simulink library "xps_library"  (R2021a)
settings: Solver=VariableStepAuto  StartTime=0.0  StopTime=10.0  RelTol=1e-3
undefined symbols (not defined in the file or in its folder): ip_name, lib_path
libraries: xbsIndex_r4 x2626, casper_library_flow_control x68, simulink x52, $bdroot x9, casper_library_misc x9
(part 5 of 33)

== system xps_library/Platforms ==
  ADM_PCIE_9H7 : Subsystem  Tag=xps:xsg  mask(xsg core config){hw_sys=ADM_PCIE_9H7:xcvu37p, clk_src=sys_clk, clk_rate=100, use_microblaze=off, use_pr=on, pr_template='', sample_period=1, synthesis_tool=XST}
      mask prompts: hw_sys "Hardware Platform"; clk_src "User IP Clock source"; clk_rate "User IP Clock Rate (MHz)"; use_microblaze "Use Microblaze controller?"; use_pr "Use PCIe Partial Reconfiguration"; sample_period "Sample Period"; synthesis_tool "Synthesis Tool:"
      mask help:
      | The XSG Core Config block is used to configure the System Generator design
      | for the casper_xps toolflow. Settings here are used to configure the
      | Xilinx System Generator block parameters automatically, and control toolflow
      | script  execution. It needs to be at the top level of all designs being compiled
      | with the casper_xps toolflow.
      mask init:
      | xps_xsg_adm_pcie_9h7_conf_mask;
      mask Help: eval('xlWeb([getenv(''MLIB_ROOT''), ''\doc\html\sys_xsg_core_config\sys_xsg_core_config.html''])')
      mask TypeOptions hw_sys: ADM_PCIE_9H7:xcvu37p
      mask TypeOptions clk_src: sys_clk | dts_clk
      mask TypeOptions synthesis_tool: Leonardo Spectrum | Synplify | Synplify Pro | XST
      mask Display: fprintf(['ADM\nPCIE_9H7']);
  AU280 : Subsystem  Tag=xps:xsg  mask(xsg core config){hw_sys=AU280:xcu280, clk_src=sys_clk, clk_rate=156.25, sample_period=1, synthesis_tool=XST}
      mask prompts: hw_sys "Hardware Platform"; clk_src "User IP Clock source"; clk_rate "User IP Clock Rate (MHz)"; sample_period "Sample Period"; synthesis_tool "Synthesis Tool:"
      mask help:
      | The XSG Core Config block is used to configure the System Generator design
      | for the casper_xps toolflow. Settings here are used to configure the
      | Xilinx System Generator block parameters automatically, and control toolflow
      | script  execution. It needs to be at the top level of all designs being compiled
      | with the casper_xps toolflow.
      mask init:
      | xps_xsg_au280_conf_mask;
      mask Help: eval('xlWeb([getenv(''MLIB_ROOT''), ''\doc\html\sys_xsg_core_config\sys_xsg_core_config.html''])')
      mask TypeOptions hw_sys: AU280:xcu280
      mask TypeOptions clk_src: sys_clk | aux_clk
      mask TypeOptions synthesis_tool: Leonardo Spectrum | Synplify | Synplify Pro | XST
      mask Display: fprintf(['ALVEO_U280']);
  AU50 : Subsystem  Tag=xps:xsg  mask(xsg core config){hw_sys=AU50:xcu50, clk_src=sys_clk, clk_rate=156.25, sample_period=1, synthesis_tool=XST}
      mask prompts: hw_sys "Hardware Platform"; clk_src "User IP Clock source"; clk_rate "User IP Clock Rate (MHz)"; sample_period "Sample Period"; synthesis_tool "Synthesis Tool:"
      mask help:
      | The XSG Core Config block is used to configure the System Generator design
      | for the casper_xps toolflow. Settings here are used to configure the
      | Xilinx System Generator block parameters automatically, and control toolflow
      | script  execution. It needs to be at the top level of all designs being compiled
      | with the casper_xps toolflow.
      mask init:
      | xps_xsg_au50_conf_mask;
      mask Help: eval('xlWeb([getenv(''MLIB_ROOT''), ''\doc\html\sys_xsg_core_config\sys_xsg_core_config.html''])')
      mask TypeOptions hw_sys: AU50:xcu50
      mask TypeOptions clk_src: sys_clk | aux_clk
      mask TypeOptions synthesis_tool: Leonardo Spectrum | Synplify | Synplify Pro | XST
      mask Display: fprintf(['ALVEO_U50']);
  CASIA_K7 : Subsystem  Tag=xps:xsg  AncestorBlock=xps_merge/Platforms/CASIA_K7  mask(xsg core config){hw_sys=CASIA_K7:xc7k325t, clk_src=sys_clk, clk_rate=100, use_microblaze=on, sample_period=1, synthesis_tool=XST}
      mask prompts: hw_sys "Hardware Platform"; clk_src "User IP Clock source"; clk_rate "User IP Clock Rate (MHz)"; use_microblaze "Use Microblaze controller?"; sample_period "Sample Period"; synthesis_tool "Synthesis Tool:"
      mask help:
      | The XSG Core Config block is used to configure the System Generator design
      | for the casper_xps toolflow. Settings here are used to configure the
      | Xilinx System Generator block parameters automatically, and control toolflow
      | script  execution. It needs to be at the top level of all designs being compiled
      | with the casper_xps toolflow.
      mask init:
      | xps_xsg_casia_k7_conf_mask;
      mask Help: eval('xlWeb([getenv(''MLIB_ROOT''), ''\doc\html\sys_xsg_core_config\sys_xsg_core_config.html''])')
      mask TypeOptions hw_sys: CASIA_K7:xc7k325t
      mask TypeOptions clk_src: sys_clk | clk_250MHz | adc_clk
      mask TypeOptions synthesis_tool: Leonardo Spectrum | Synplify | Synplify Pro | XST
      mask Display: fprintf(['CASIA_K7']);
  CASIA_K7_21CMA : Subsystem  Tag=xps:xsg  AncestorBlock=xps_merge/Platforms/CASIA_K7_21CMA  mask(xsg core config){hw_sys=CASIA_K7_21CMA:xc7k325t, clk_src=sys_clk, clk_rate=100, use_microblaze=on, sample_period=1, synthesis_tool=XST}
      mask prompts: hw_sys "Hardware Platform"; clk_src "User IP Clock source"; clk_rate "User IP Clock Rate (MHz)"; use_microblaze "Use Microblaze controller?"; sample_period "Sample Period"; synthesis_tool "Synthesis Tool:"
      mask help:
      | The XSG Core Config block is used to configure the System Generator design
      | for the casper_xps toolflow. Settings here are used to configure the
      | Xilinx System Generator block parameters automatically, and control toolflow
      | script  execution. It needs to be at the top level of all designs being compiled
      | with the casper_xps toolflow.
      mask init:
      | xps_xsg_casia_k7_21cma_conf_mask;
      mask Help: eval('xlWeb([getenv(''MLIB_ROOT''), ''\doc\html\sys_xsg_core_config\sys_xsg_core_config.html''])')
      mask TypeOptions hw_sys: CASIA_K7_21CMA:xc7k325t
      mask TypeOptions clk_src: sys_clk | clk_250MHz | adc_clk
      mask TypeOptions synthesis_tool: Leonardo Spectrum | Synplify | Synplify Pro | XST
      mask Display: fprintf(['CASIA_K7_21CMA']);
  HTG9200 : Subsystem  Tag=xps:xsg  mask(xsg core config){hw_sys=HTG9200:xcvu13p, clk_src=sys_clk, clk_rate=100, use_microblaze=on, sample_period=1, synthesis_tool=XST}
      mask prompts: hw_sys "Hardware Platform"; clk_src "User IP Clock source"; clk_rate "User IP Clock Rate (MHz)"; use_microblaze "Use Microblaze controller?"; sample_period "Sample Period"; synthesis_tool "Synthesis Tool:"
      mask help:
      | The XSG Core Config block is used to configure the System Generator design
      | for the casper_xps toolflow. Settings here are used to configure the
      | Xilinx System Generator block parameters automatically, and control toolflow
      | script  execution. It needs to be at the top level of all designs being compiled
      | with the casper_xps toolflow.
      mask init:
      | xps_xsg_htg9200_conf_mask;
      mask Help: eval('xlWeb([getenv(''MLIB_ROOT''), ''\doc\html\sys_xsg_core_config\sys_xsg_core_config.html''])')
      mask TypeOptions hw_sys: HTG9200:xcvu13p
      mask TypeOptions clk_src: sys_clk | clk_250
      mask TypeOptions synthesis_tool: Leonardo Spectrum | Synplify | Synplify Pro | XST
      mask Display: fprintf(['HTG9200']);
  HTG940 : Subsystem  Tag=xps:xsg  mask(xsg core config){hw_sys=HTG940:xcvu13p, clk_src=fmc_c_clk, clk_rate=312.5, use_microblaze=on, sample_period=1, synthesis_tool=XST}
      mask prompts: hw_sys "Hardware Platform"; clk_src "User IP Clock source"; clk_rate "User IP Clock Rate (MHz)"; use_microblaze "Use Microblaze controller?"; sample_period "Sample Period"; synthesis_tool "Synthesis Tool:"
      mask help:
      | The XSG Core Config block is used to configure the System Generator design
      | for the casper_xps toolflow. Settings here are used to configure the
      | Xilinx System Generator block parameters automatically, and control toolflow
      | script  execution. It needs to be at the top level of all designs being compiled
      | with the casper_xps toolflow.
      mask init:
      | xps_xsg_htg940_conf_mask;
      mask Help: eval('xlWeb([getenv(''MLIB_ROOT''), ''\doc\html\sys_xsg_core_config\sys_xsg_core_config.html''])')
      mask TypeOptions hw_sys: HTG940:xcvu13p
      mask TypeOptions clk_src: sys_clk | fmc_a_clk | fmc_b_clk | fmc_c_clk | fmc_d_clk | ddr_refclk
      mask TypeOptions synthesis_tool: Leonardo Spectrum | Synplify | Synplify Pro | XST
      mask Display: fprintf(['HTG940']);
  HTG_ZRF16 : Subsystem  Tag=xps:xsg  mask(xsg core config){hw_sys=htg_zrf16:xczu49dr, clk_src=sys_clk, clk_rate=100, sample_period=1, synthesis_tool=XST}
      mask prompts: hw_sys "Hardware Platform"; clk_src "User IP Clock source"; clk_rate "User IP Clock Rate (MHz)"; sample_period "Sample Period"; synthesis_tool "Synthesis Tool:"
      mask help:
      | The XSG Core Config block is used to configure the System Generator design
      | for the casper_xps toolflow. Settings here are used to configure the
      | Xilinx System Generator block parameters automatically, and control toolflow
      | script  execution. It needs to be at the top level of all designs being compiled
      | with the casper_xps toolflow.
      mask init:
      | xps_xsg_htg_zrf16_conf_mask;
      mask Help: eval('xlWeb([getenv(''MLIB_ROOT''), ''\doc\html\sys_xsg_core_config\sys_xsg_core_config.html''])')
      mask TypeOptions hw_sys: htg_zrf16:xczu29dr | htg_zrf16:xczu49dr
      mask TypeOptions clk_src: sys_clk | adc_clk | arb_clk
      mask TypeOptions synthesis_tool: Leonardo Spectrum | Synplify | Synplify Pro | XST
      mask Display: fprintf(['ZRF16']);
  MX175 : Subsystem  Tag=xps:xsg  mask(xsg core config){hw_sys=MX175:xc7vx690t, clk_src=sys_clk, clk_rate=100, use_microblaze=off, sample_period=1, synthesis_tool=XST}
      mask prompts: hw_sys "Hardware Platform"; clk_src "User IP Clock source"; clk_rate "User IP Clock Rate (MHz)"; use_microblaze "Use Microblaze controller?"; sample_period "Sample Period"; synthesis_tool "Synthesis Tool:"
      mask help:
      | The XSG Core Config block is used to configure the System Generator design
      | for the casper_xps toolflow. Settings here are used to configure the
      | Xilinx System Generator block parameters automatically, and control toolflow
      | script  execution. It needs to be at the top level of all designs being compiled
      | with the casper_xps toolflow.
      mask init:
      | xps_xsg_mx175_conf_mask;
      mask Help: eval('xlWeb([getenv(''MLIB_ROOT''), ''\doc\html\sys_xsg_core_config\sys_xsg_core_config.html''])')
      mask TypeOptions hw_sys: MX175:xc7vx690t
      mask TypeOptions clk_src: sys_clk | adc0_clk
      mask TypeOptions synthesis_tool: Leonardo Spectrum | Synplify | Synplify Pro | XST
      mask Display: fprintf(['MX175']);
  RED_PITAYA : Subsystem  Tag=xps:xsg  mask(xsg core config){hw_sys=RED_PITAYA_10:xc7z010, clk_src=sys_clk, clk_rate=125, sample_period=1, synthesis_tool=XST}
      mask prompts: hw_sys "Hardware Platform"; clk_src "User IP Clock source"; clk_rate "User IP Clock Rate (MHz)"; sample_period "Sample Period"; synthesis_tool "Synthesis Tool:"
      mask help:
      | The XSG Core Config block is used to configure the System Generator design
      | for the casper_xps toolflow. Settings here are used to configure the
      | Xilinx System Generator block parameters automatically, and control toolflow
      | script  execution. It needs to be at the top level of all designs being compiled
      | with the casper_xps toolflow.
      mask init:
      | xps_xsg_red_pitaya_conf_mask;
      mask Help: eval('xlWeb([getenv(''MLIB_ROOT''), ''\doc\html\sys_xsg_core_config\sys_xsg_core_config.html''])')
      mask TypeOptions hw_sys: RED_PITAYA_10:xc7z010 | RED_PITAYA_14:xc7z010
      mask TypeOptions clk_src: sys_clk | adc_clk
      mask Callback clk_src: xps_xsg_red_pitaya_conf_mask_callback;
      mask TypeOptions synthesis_tool: Leonardo Spectrum | Synplify | Synplify Pro | XST
      mask Display: fprintf(['RED_PITAYA']);
  RFSoC2x2 : Subsystem  Tag=xps:xsg  AncestorBlock=xps_library/Platforms/PYNQ2x2  mask(xsg core config){hw_sys=rfsoc2x2:xczu28dr, clk_src=adc_clk, clk_rate=245.76, pl_clk_rate=122.88, sample_period=1, synthesis_tool=XST}
      mask prompts: hw_sys "Hardware Platform"; clk_src "User IP Clock source"; clk_rate "User IP Clock Rate (MHz)"; pl_clk_rate "RFPLL PL Clock Rate (MHz)"; sample_period "Sample Period"; synthesis_tool "Synthesis Tool:"
      mask help:
      | The XSG Core Config block is used to configure the System Generator design
      | for the casper_xps toolflow. Settings here are used to configure the
      | Xilinx System Generator block parameters automatically, and control toolflow
      | script  execution. It needs to be at the top level of all designs being compiled
      | with the casper_xps toolflow.
      mask init:
      | xps_xsg_rfsoc2x2_conf_mask;
      mask Help: eval('xlWeb([getenv(''MLIB_ROOT''), ''\doc\html\sys_xsg_core_config\sys_xsg_core_config.html''])')
      mask TypeOptions hw_sys: rfsoc2x2:xczu28dr
      mask TypeOptions clk_src: adc_clk
      mask TypeOptions synthesis_tool: Leonardo Spectrum | Synplify | Synplify Pro | XST
      mask Display: fprintf(['RFSoC2x2']);
  RFSoC4x2 : Subsystem  Tag=xps:xsg  AncestorBlock=xps_library/Platforms/ZCU216  mask(xsg core config){hw_sys=rfsoc4x2:xczu48dr, clk_src=adc_clk, clk_rate=245.76, pl_clk_rate=122.88, sample_period=1, synthesis_tool=XST}
      mask prompts: hw_sys "Hardware Platform"; clk_src "User IP Clock source"; clk_rate "User IP Clock Rate (MHz)"; pl_clk_rate "RFPLL PL Clock Rate (MHz)"; sample_period "Sample Period"; synthesis_tool "Synthesis Tool:"
      mask help:
      | The XSG Core Config block is used to configure the System Generator design
      | for the casper_xps toolflow. Settings here are used to configure the
      | Xilinx System Generator block parameters automatically, and control toolflow
      | script  execution. It needs to be at the top level of all designs being compiled
      | with the casper_xps toolflow.
      mask init:
      | xps_xsg_rfsoc4x2_conf_mask;
      mask Help: eval('xlWeb([getenv(''MLIB_ROOT''), ''\doc\html\sys_xsg_core_config\sys_xsg_core_config.html''])')
      mask TypeOptions hw_sys: rfsoc4x2:xczu48dr
      mask TypeOptions clk_src: adc_clk
      mask TypeOptions synthesis_tool: Leonardo Spectrum | Synplify | Synplify Pro | XST
      mask Display: fprintf(['RFSoC4x2']);
  SKARAB : Subsystem  Tag=xps:xsg  mask(xsg core config){hw_sys=SKARAB:xc7vx690t, clk_src=adc_clk, clk_rate=230, sample_period=1, synthesis_tool=XST}
      mask prompts: hw_sys "Hardware Platform"; clk_src "User IP Clock source"; clk_rate "User IP Clock Rate (MHz)"; sample_period "Sample Period"; synthesis_tool "Synthesis Tool:"
      mask help:
      | The XSG Core Config block is used to configure the System Generator design
      | for the casper_xps toolflow. Settings here are used to configure the
      | Xilinx System Generator block parameters automatically, and control toolflow
      | script  execution. It needs to be at the top level of all designs being compiled
      | with the casper_xps toolflow.
      mask init:
      | xps_xsg_skarab_conf_mask;
      mask Help: eval('xlWeb([getenv(''MLIB_ROOT''), ''\doc\html\sys_xsg_core_config\sys_xsg_core_config.html''])')
      mask TypeOptions hw_sys: SKARAB:xc7vx690t
      mask TypeOptions clk_src: sys_clk | adc_clk | aux_clk
      mask Callback clk_src: xps_xsg_skarab_conf_mask_callback
      mask TypeOptions synthesis_tool: Leonardo Spectrum | Synplify | Synplify Pro | XST
      mask Display: fprintf(['SKARAB']);
  SNAP : Subsystem  Tag=xps:xsg  mask(xsg core config){hw_sys=SNAP:xc7k160t, clk_src=sys_clk, clk_rate=100, use_microblaze=off, sample_period=1, synthesis_tool=XST}
      mask prompts: hw_sys "Hardware Platform"; clk_src "User IP Clock source"; clk_rate "User IP Clock Rate (MHz)"; use_microblaze "Use Microblaze controller?"; sample_period "Sample Period"; synthesis_tool "Synthesis Tool:"
      mask help:
      | The XSG Core Config block is used to configure the System Generator design
      | for the casper_xps toolflow. Settings here are used to configure the
      | Xilinx System Generator block parameters automatically, and control toolflow
      | script  execution. It needs to be at the top level of all designs being compiled
      | with the casper_xps toolflow.
      mask init:
      | xps_xsg_snap_conf_mask;
      mask Help: eval('xlWeb([getenv(''MLIB_ROOT''), ''\doc\html\sys_xsg_core_config\sys_xsg_core_config.html''])')
      mask TypeOptions hw_sys: SNAP:xc7k160t
      mask TypeOptions clk_src: sys_clk | adc0_clk
      mask TypeOptions synthesis_tool: Leonardo Spectrum | Synplify | Synplify Pro | XST
      mask Display: fprintf(['SNAP']);
  SNAP2 : Subsystem  Tag=xps:xsg  mask(xsg core config){hw_sys=SNAP2_v1:xcku115, clk_src=adc0_clk, clk_rate=250, use_microblaze=off, sample_period=1, synthesis_tool=XST}
      mask prompts: hw_sys "Hardware Platform"; clk_src "User IP Clock source"; clk_rate "User IP Clock Rate (MHz)"; use_microblaze "Use Microblaze controller?"; sample_period "Sample Period"; synthesis_tool "Synthesis Tool:"
      mask help:
      | The XSG Core Config block is used to configure the System Generator design
      | for the casper_xps toolflow. Settings here are used to configure the
      | Xilinx System Generator block parameters automatically, and control toolflow
      | script  execution. It needs to be at the top level of all designs being compiled
      | with the casper_xps toolflow.
      mask init:
      | xps_xsg_snap2_conf_mask;
      mask Help: eval('xlWeb([getenv(''MLIB_ROOT''), ''\doc\html\sys_xsg_core_config\sys_xsg_core_config.html''])')
      mask TypeOptions hw_sys: SNAP2_v1:xcku115 | SNAP2_v2:xcku115
      mask TypeOptions clk_src: sys_clk | clk_250MHz | adc0_clk | adc1_clk | clk_200
      mask TypeOptions synthesis_tool: Leonardo Spectrum | Synplify | Synplify Pro | XST
      mask Display: fprintf(['SNAP2']);
  SPARROW : Subsystem  Tag=xps:xsg  AncestorBlock=xps_library/Platforms/SPARROW  mask(xsg core config){hw_sys=SPARROW:xc7z030, clk_src=sys_clk, clk_rate=100, use_sfp_ethernet=on, another_sfp=on, sample_period=1, synthesis_tool=XST}
      mask prompts: hw_sys "Hardware Platform"; clk_src "User IP Clock source"; clk_rate "User IP Clock Rate (MHz)"; use_sfp_ethernet "Use SFP Ethernet (Do this for boards with buggy RJ45!)"; another_sfp "Use SFP3 (only allowed if there is a 1GbE port on SFP 0)"; sample_period "Sample Period"; synthesis_tool "Synthesis Tool:"
      mask help:
      | The XSG Core Config block is used to configure the System Generator design
      | for the casper_xps toolflow. Settings here are used to configure the
      | Xilinx System Generator block parameters automatically, and control toolflow
      | script  execution. It needs to be at the top level of all designs being compiled
      | with the casper_xps toolflow.
      mask init:
      | xps_xsg_sparrow_conf_mask;
      mask Help: eval('xlWeb([getenv(''MLIB_ROOT''), ''\doc\html\sys_xsg_core_config\sys_xsg_core_config.html''])')
      mask TypeOptions hw_sys: SPARROW:xc7z030 | SPARROW:xc7z035 | SPARROW:xc7z045
      mask TypeOptions clk_src: sys_clk | adc_clk
      mask TypeOptions synthesis_tool: Leonardo Spectrum | Synplify | Synplify Pro | XST
      mask Display: fprintf(['SPARROW']);
  VCU118 : Subsystem  Tag=xps:xsg  mask(xsg core config){hw_sys=VCU118:xcvu9p, clk_src=clk_200mhz, clk_rate=200, axi_master=jtag, sample_period=1, synthesis_tool=XST}
      mask prompts: hw_sys "Hardware Platform"; clk_src "User IP Clock source"; clk_rate "User IP Clock Rate (MHz)"; axi_master "Which type of control interface?"; sample_period "Sample Period"; synthesis_tool "Synthesis Tool:"
      mask help:
      | The XSG Core Config block is used to configure the System Generator design
      | for the casper_xps toolflow. Settings here are used to configure the
      | Xilinx System Generator block parameters automatically, and control toolflow
      | script  execution. It needs to be at the top level of all designs being compiled
      | with the casper_xps toolflow.
      mask init:
      | xps_xsg_vcu118_conf_mask;
      mask Help: eval('xlWeb([getenv(''MLIB_ROOT''), ''\doc\html\sys_xsg_core_config\sys_xsg_core_config.html''])')
      mask TypeOptions hw_sys: VCU118:xcvu9p
      mask TypeOptions clk_src: sys_clk | clk_200mhz
      mask TypeOptions axi_master: microblaze | pci | spi | jtag
      mask TypeOptions synthesis_tool: Leonardo Spectrum | Synplify | Synplify Pro | XST
      mask Display: fprintf(['VCU118']);
  VCU128 : Subsystem  Tag=xps:xsg  mask(xsg core config){hw_sys=VCU128:xcvu37p, clk_src=sys_clk, clk_rate=100, use_microblaze=on, sample_period=1, synthesis_tool=XST}
      mask prompts: hw_sys "Hardware Platform"; clk_src "User IP Clock source"; clk_rate "User IP Clock Rate (MHz)"; use_microblaze "Use Microblaze controller?"; sample_period "Sample Period"; synthesis_tool "Synthesis Tool:"
      mask help:
      | The XSG Core Config block is used to configure the System Generator design
      | for the casper_xps toolflow. Settings here are used to configure the
      | Xilinx System Generator block parameters automatically, and control toolflow
      | script  execution. It needs to be at the top level of all designs being compiled
      | with the casper_xps toolflow.
      mask init:
      | xps_xsg_vcu128_conf_mask;
      mask Help: eval('xlWeb([getenv(''MLIB_ROOT''), ''\doc\html\sys_xsg_core_config\sys_xsg_core_config.html''])')
      mask TypeOptions hw_sys: VCU128:xcvu37p
      mask TypeOptions clk_src: sys_clk | adc_clk
      mask TypeOptions synthesis_tool: Leonardo Spectrum | Synplify | Synplify Pro | XST
      mask Display: fprintf(['VCU128']);
  ZCU111 : Subsystem  Tag=xps:xsg  mask(xsg core config){hw_sys=ZCU111:xczu28dr, clk_src=adc_clk, clk_rate=250, pl_clk_rate=125, sample_period=1, synthesis_tool=XST}
      mask prompts: hw_sys "Hardware Platform"; clk_src "User IP Clock source"; clk_rate "User IP Clock Rate (MHz)"; pl_clk_rate "RFPLL PL Clock Rate (MHz)"; sample_period "Sample Period"; synthesis_tool "Synthesis Tool:"
      mask help:
      | The XSG Core Config block is used to configure the System Generator design
      | for the casper_xps toolflow. Settings here are used to configure the
      | Xilinx System Generator block parameters automatically, and control toolflow
      | script  execution. It needs to be at the top level of all designs being compiled
      | with the casper_xps toolflow.
      mask init:
      | xps_xsg_zcu111_conf_mask;
      mask Help: eval('xlWeb([getenv(''MLIB_ROOT''), ''\doc\html\sys_xsg_core_config\sys_xsg_core_config.html''])')
      mask TypeOptions hw_sys: ZCU111:xczu28dr
      mask TypeOptions clk_src: adc_clk
      mask TypeOptions synthesis_tool: Leonardo Spectrum | Synplify | Synplify Pro | XST
      mask Display: fprintf(['ZCU111']);
  ZCU208 : Subsystem  Tag=xps:xsg  mask(xsg core config){hw_sys=ZCU208:xczu48dr, clk_src=adc_clk, clk_rate=250, pl_clk_rate=125, sample_period=1, synthesis_tool=XST}
      mask prompts: hw_sys "Hardware Platform"; clk_src "User IP Clock source"; clk_rate "User IP Clock Rate (MHz)"; pl_clk_rate "RFPLL PL Clock Rate (MHz)"; sample_period "Sample Period"; synthesis_tool "Synthesis Tool:"
      mask help:
      | The XSG Core Config block is used to configure the System Generator design
      | for the casper_xps toolflow. Settings here are used to configure the
      | Xilinx System Generator block parameters automatically, and control toolflow
      | script  execution. It needs to be at the top level of all designs being compiled
      | with the casper_xps toolflow.
      mask init:
      | xps_xsg_zcu208_conf_mask;
      mask Help: eval('xlWeb([getenv(''MLIB_ROOT''), ''\doc\html\sys_xsg_core_config\sys_xsg_core_config.html''])')
      mask TypeOptions hw_sys: ZCU208:xczu48dr
      mask TypeOptions clk_src: adc_clk
      mask TypeOptions synthesis_tool: Leonardo Spectrum | Synplify | Synplify Pro | XST
      mask Display: fprintf(['ZCU208']);
  ZCU216 : Subsystem  Tag=xps:xsg  mask(xsg core config){hw_sys=ZCU216:xczu49dr, clk_src=adc_clk, clk_rate=250, pl_clk_rate=125, sample_period=1, synthesis_tool=XST}
      mask prompts: hw_sys "Hardware Platform"; clk_src "User IP Clock source"; clk_rate "User IP Clock Rate (MHz)"; pl_clk_rate "RFPLL PL Clock Rate (MHz)"; sample_period "Sample Period"; synthesis_tool "Synthesis Tool:"
      mask help:
      | The XSG Core Config block is used to configure the System Generator design
      | for the casper_xps toolflow. Settings here are used to configure the
      | Xilinx System Generator block parameters automatically, and control toolflow
      | script  execution. It needs to be at the top level of all designs being compiled
      | with the casper_xps toolflow.
      mask init:
      | xps_xsg_zcu216_conf_mask;
      mask Help: eval('xlWeb([getenv(''MLIB_ROOT''), ''\doc\html\sys_xsg_core_config\sys_xsg_core_config.html''])')
      mask TypeOptions hw_sys: ZCU216:xczu49dr
      mask TypeOptions clk_src: adc_clk
      mask TypeOptions synthesis_tool: Leonardo Spectrum | Synplify | Synplify Pro | XST
      mask Display: fprintf(['ZCU216']);
  ZRF16 : Subsystem  Tag=xps:xsg  mask(xsg core config){hw_sys=ZRF16_49DR:xczu49dr, clk_src=adc_clk, clk_rate=250, pl_clk_rate=125, sample_period=1, synthesis_tool=XST}
      mask prompts: hw_sys "Hardware Platform"; clk_src "User IP Clock source"; clk_rate "User IP Clock Rate (MHz)"; pl_clk_rate "RFPLL PL Clock Rate (MHz)"; sample_period "Sample Period"; synthesis_tool "Synthesis Tool:"
      mask help:
      | The XSG Core Config block is used to configure the System Generator design
      | for the casper_xps toolflow. Settings here are used to configure the
      | Xilinx System Generator block parameters automatically, and control toolflow
      | script  execution. It needs to be at the top level of all designs being compiled
      | with the casper_xps toolflow.
      mask init:
      | xps_xsg_zrf16_conf_mask;
      mask Help: eval('xlWeb([getenv(''MLIB_ROOT''), ''\doc\html\sys_xsg_core_config\sys_xsg_core_config.html''])')
      mask TypeOptions hw_sys: ZRF16_49DR:xczu49dr | ZRF16_29DR:xczu29dr
      mask TypeOptions clk_src: adc_clk
      mask TypeOptions synthesis_tool: Leonardo Spectrum | Synplify | Synplify Pro | XST
      mask Display: fprintf(['ZRF16']);

== system xps_library/Utilities ==
  dcp : Subsystem  Tag=xps:dcp  mask(ip){dcp_file=}
      mask prompts: dcp_file "Name of the DCP file"
      mask help: Allows insertion of custom Xilinx IP content from user created libraries.
      mask Display: fprintf('DCP');
  exception_constraint : Subsystem  Tag=xps:exception_constr  mask(exception_constraint){constraint_type=Multicycle Constraint, num_clock_cycles=4}
      mask prompts: constraint_type "Constraint Type"; num_clock_cycles "Number of Clock Cycles"
      mask help: Yellow Block utility to add to a signal path to be marked with a False Path or Multicycle constraint.
      mask init:
      | exception_constr_mask;
      mask Help:
      | For more information, please see Xilinx's Constraints User Guide at the link below, page 106:
      | - https://www.xilinx.com/support/documentation/sw_manuals/xilinx2018_1/ug903-vivado-using-constraints.pdf
      mask TypeOptions constraint_type: False Path Constraint | Multicycle Constraint
      mask Callback constraint_type:
      | mask_enables = get_param(gcb, 'MaskEnables');
      | mask_names = get_param(gcb, 'MaskNames');
      | if strcmp(get_param(gcb, 'constraint_type'), 'False Path Constraint'),
      |     mask_enables{ismember(mask_names, 'num_clock_cycles')} = 'off';
      | else
      |     mask_enables{ismember(mask_names, 'num_clock_cycles')} = 'on';
      | end
      | set_param(gcb, 'MaskEnables', mask_enables);
  ip : Subsystem  Tag=xps:ip  mask(ip){lib_path=lib_path, ip_name=ip_name}
      mask prompts: lib_path "Path to sysgen build directory (the directory containing ip/)"; ip_name "Name of IP in this library"
      mask help: Allows insertion of custom Xilinx IP content from user created libraries.
      mask Display: fprintf('IP');
  white_rabbit : Subsystem  Tag=xps:white_rabbit  mask(white_rabbit){}
      mask help: Instantiates a White Rabbit timing recovery core
      mask init:
      | white_rabbit_init(gcb)
      mask Display: fprintf('WHITE\nRABBIT');

== system xps_library/ADCs/adc ==
  sim_in : Inport  SampleTime=sample_period/4
  sim_sync : Inport  Port=2  SampleTime=sample_period/4
  sim_data_valid : Inport  Port=3  SampleTime=sample_period/4
  Compare To Constant{,1..2,5,8..10,13} (8 alike) : simulink/Logic and Bit Operations/Compare To Constant  relop=>  const=255  OutDataTypeStr=boolean  ZeroCross=off
  Compare To Constant{3..4,6..7,11..12,14..15} (8 alike) : simulink/Logic and Bit Operations/Compare To Constant  relop=<  const=0  OutDataTypeStr=boolean  ZeroCross=off
  Logical Operator{,1..3} (4 alike) : Logic  Operator=OR  Inputs=4  AllPortsSameDT=off  OutDataTypeStr=boolean
  bias : Bias  Bias=127.5  SaturateOnIntegerOverflow=on
  conv : Subsystem
  conv1 : Subsystem
  conv2 : Subsystem
  conv3 : Subsystem
  conv4 : Subsystem
  conv5 : Subsystem
  conv6 : Subsystem
  conv7 : Subsystem
  delayi{0..3,7,11,13} (7 alike) : Delay  DelayLength=1
  delayi10 : Delay
  delayi12 : Delay
  delayi14 : Delay  DelayLength=4
  delayi15 : Delay  DelayLength=3
  delayi4 : Delay  DelayLength=4
  delayi5 : Delay  DelayLength=3
  delayi6 : Delay
  delayi8 : Delay  DelayLength=4
  delayi9 : Delay  DelayLength=3
  delayq{0..3} (4 alike) : Delay  DelayLength=1
  delaysync0 : Delay
  delaysync1 : Delay  DelayLength=1
  delaysync2 : Delay  DelayLength=1
  delaysync3 : Delay  DelayLength=1
  gain : Gain  Gain=127.5  SaturateOnIntegerOverflow=on  OutDataTypeStr=Inherit: Same as input  ParamDataTypeStr=Inherit: Same as input
  xps_library_ADCs_adc_user_data_valid : xbsIndex_r4/Gateway In  gui_display_data_type=Fixed-point  arith_type=Boolean  n_bits=8  bin_pt=0  preci_type=Single  exp_width=8  frac_width=24  rows=1  columns=1  quantization="Round  (unbiased: +/- Inf)"  overflow=Saturate  period=sample_period  UseAsADC=off  ADCChannel='1'  interface=None  automatic_assignment=on  address_offset=hex2dec('00')  intf_name=''  intf_description=''  default_value=0  timing_constraint=None  locs_specified=off  LOCs={}  io_standard={}  inherit_from_input=off  hdl_port=on  dbl_ovrd=off  block_type=gatewayin
      settings: infoedit="Gateway in block.  Converts inputs of type Simulink integer, double and fixed point to  Xilinx fixed point type.<P><P>Hardware notes:  In hardware these blocks become top level input ports."  xl_area=[0 0 0 0 8 0 0]  block_version=8.2.02
  xps_library_ADCs_adc_user_datai{0..3} (4 alike) : xbsIndex_r4/Gateway In  gui_display_data_type=Fixed-point  arith_type=Unsigned  n_bits=8  bin_pt=0  preci_type=Single  exp_width=8  frac_width=24  rows=1  columns=1  quantization="Round  (unbiased: +/- Inf)"  overflow=Saturate  period=sample_period  UseAsADC=off  ADCChannel='1'  interface=None  automatic_assignment=on  address_offset=hex2dec('00')  intf_name=''  intf_description=''  default_value=0  timing_constraint=None  locs_specified=off  LOCs={}  io_standard={}  inherit_from_input=off  hdl_port=on  dbl_ovrd=off  block_type=gatewayin
      settings: infoedit="Gateway in block.  Converts inputs of type Simulink integer, double and fixed point to  Xilinx fixed point type.<P><P>Hardware notes:  In hardware these blocks become top level input ports."  xl_area=[0 0 0 0 8 0 0]  block_version=8.2.02
  xps_library_ADCs_adc_user_dataq{0..3} (4 alike) : xbsIndex_r4/Gateway In  gui_display_data_type=Fixed-point  arith_type=Unsigned  n_bits=8  bin_pt=0  preci_type=Single  exp_width=8  frac_width=24  rows=1  columns=1  quantization="Round  (unbiased: +/- Inf)"  overflow=Saturate  period=sample_period  UseAsADC=off  ADCChannel='1'  interface=None  automatic_assignment=on  address_offset=hex2dec('00')  intf_name=''  intf_description=''  default_value=0  timing_constraint=None  locs_specified=off  LOCs={}  io_standard={}  inherit_from_input=off  hdl_port=on  dbl_ovrd=off  block_type=gatewayin
      settings: infoedit="Gateway in block.  Converts inputs of type Simulink integer, double and fixed point to  Xilinx fixed point type.<P><P>Hardware notes:  In hardware these blocks become top level input ports."  xl_area=[0 0 0 0 8 0 0]  block_version=8.2.02
  xps_library_ADCs_adc_user_outofrangei0 : xbsIndex_r4/Gateway In  gui_display_data_type=Fixed-point  arith_type=Boolean  n_bits=8  bin_pt=0  preci_type=Single  exp_width=8  frac_width=24  rows=1  columns=1  quantization="Round  (unbiased: +/- Inf)"  overflow=Saturate  period=sample_period  UseAsADC=off  ADCChannel='1'  interface=None  automatic_assignment=on  address_offset=hex2dec('00')  intf_name=''  intf_description=''  default_value=0  timing_constraint=None  locs_specified=off  LOCs={}  io_standard={}  inherit_from_input=off  hdl_port=on  dbl_ovrd=off  block_type=gatewayin
      settings: infoedit="Gateway in block.  Converts inputs of type Simulink integer, double and fixed point to  Xilinx fixed point type.<P><P>Hardware notes:  In hardware these blocks become top level input ports."  xl_area=[0 0 0 0 8 0 0]  block_version=8.2.02
  xps_library_ADCs_adc_user_outofrangei1 : xbsIndex_r4/Gateway In  gui_display_data_type=Fixed-point  arith_type=Boolean  n_bits=8  bin_pt=0  preci_type=Single  exp_width=8  frac_width=24  rows=1  columns=1  quantization="Round  (unbiased: +/- Inf)"  overflow=Saturate  period=sample_period  UseAsADC=off  ADCChannel='1'  interface=None  automatic_assignment=on  address_offset=hex2dec('00')  intf_name=''  intf_description=''  default_value=0  timing_constraint=None  locs_specified=off  LOCs={}  io_standard={}  inherit_from_input=off  hdl_port=on  dbl_ovrd=off  block_type=gatewayin
      settings: infoedit="Gateway in block.  Converts inputs of type Simulink integer, double and fixed point to  Xilinx fixed point type.<P><P>Hardware notes:  In hardware these blocks become top level input ports."  xl_area=[0 0 0 0 8 0 0]  block_version=8.2.02
  xps_library_ADCs_adc_user_outofrangeq0 : xbsIndex_r4/Gateway In  gui_display_data_type=Fixed-point  arith_type=Boolean  n_bits=8  bin_pt=0  preci_type=Single  exp_width=8  frac_width=24  rows=1  columns=1  quantization="Round  (unbiased: +/- Inf)"  overflow=Saturate  period=sample_period  UseAsADC=off  ADCChannel='1'  interface=None  automatic_assignment=on  address_offset=hex2dec('00')  intf_name=''  intf_description=''  default_value=0  timing_constraint=None  locs_specified=off  LOCs={}  io_standard={}  inherit_from_input=off  hdl_port=on  dbl_ovrd=off  block_type=gatewayin
      settings: infoedit="Gateway in block.  Converts inputs of type Simulink integer, double and fixed point to  Xilinx fixed point type.<P><P>Hardware notes:  In hardware these blocks become top level input ports."  xl_area=[0 0 0 0 8 0 0]  block_version=8.2.02
  xps_library_ADCs_adc_user_outofrangeq1 : xbsIndex_r4/Gateway In  gui_display_data_type=Fixed-point  arith_type=Boolean  n_bits=8  bin_pt=0  preci_type=Single  exp_width=8  frac_width=24  rows=1  columns=1  quantization="Round  (unbiased: +/- Inf)"  overflow=Saturate  period=sample_period  UseAsADC=off  ADCChannel='1'  interface=None  automatic_assignment=on  address_offset=hex2dec('00')  intf_name=''  intf_description=''  default_value=0  timing_constraint=None  locs_specified=off  LOCs={}  io_standard={}  inherit_from_input=off  hdl_port=on  dbl_ovrd=off  block_type=gatewayin
      settings: infoedit="Gateway in block.  Converts inputs of type Simulink integer, double and fixed point to  Xilinx fixed point type.<P><P>Hardware notes:  In hardware these blocks become top level input ports."  xl_area=[0 0 0 0 8 0 0]  block_version=8.2.02
  xps_library_ADCs_adc_user_sync{0..3} (4 alike) : xbsIndex_r4/Gateway In  gui_display_data_type=Fixed-point  arith_type=Boolean  n_bits=8  bin_pt=0  preci_type=Single  exp_width=8  frac_width=24  rows=1  columns=1  quantization="Round  (unbiased: +/- Inf)"  overflow=Saturate  period=sample_period  UseAsADC=off  ADCChannel='1'  interface=None  automatic_assignment=on  address_offset=hex2dec('00')  intf_name=''  intf_description=''  default_value=0  timing_constraint=None  locs_specified=off  LOCs={}  io_standard={}  inherit_from_input=off  hdl_port=on  dbl_ovrd=off  block_type=gatewayin
      settings: infoedit="Gateway in block.  Converts inputs of type Simulink integer, double and fixed point to  Xilinx fixed point type.<P><P>Hardware notes:  In hardware these blocks become top level input ports."  xl_area=[0 0 0 0 8 0 0]  block_version=8.2.02
  i0 : Outport  VectorParamsAs1DForOutWhenUnconnected=off
  i1 : Outport  Port=2  VectorParamsAs1DForOutWhenUnconnected=off
  i2 : Outport  Port=3  VectorParamsAs1DForOutWhenUnconnected=off
  i3 : Outport  Port=4  VectorParamsAs1DForOutWhenUnconnected=off
  q0 : Outport  Port=5  VectorParamsAs1DForOutWhenUnconnected=off
  q1 : Outport  Port=6  VectorParamsAs1DForOutWhenUnconnected=off
  q2 : Outport  Port=7  VectorParamsAs1DForOutWhenUnconnected=off
  q3 : Outport  Port=8  VectorParamsAs1DForOutWhenUnconnected=off
  outofrangei0 : Outport  Port=9  VectorParamsAs1DForOutWhenUnconnected=off
  outofrangei1 : Outport  Port=10  VectorParamsAs1DForOutWhenUnconnected=off
  outofrangeq0 : Outport  Port=11  VectorParamsAs1DForOutWhenUnconnected=off
  outofrangeq1 : Outport  Port=12  VectorParamsAs1DForOutWhenUnconnected=off
  sync0 : Outport  Port=13  VectorParamsAs1DForOutWhenUnconnected=off
  sync1 : Outport  Port=14  VectorParamsAs1DForOutWhenUnconnected=off
  sync2 : Outport  Port=15  VectorParamsAs1DForOutWhenUnconnected=off
  sync3 : Outport  Port=16  VectorParamsAs1DForOutWhenUnconnected=off
  data_valid : Outport  Port=17  VectorParamsAs1DForOutWhenUnconnected=off
  wires:
  delaysync1/1 -> xps_library_ADCs_adc_user_sync1/1
  delayq3/1 -> xps_library_ADCs_adc_user_dataq3/1, Compare To Constant15/1, Compare To Constant13/1
  delayq2/1 -> xps_library_ADCs_adc_user_dataq2/1, Compare To Constant14/1, Compare To Constant9/1
  delayq1/1 -> xps_library_ADCs_adc_user_dataq1/1, Compare To Constant12/1, Compare To Constant10/1
  delayi3/1 -> xps_library_ADCs_adc_user_datai3/1, Compare To Constant7/1, Compare To Constant5/1
  delayi2/1 -> xps_library_ADCs_adc_user_datai2/1, Compare To Constant6/1, Compare To Constant1/1
  delayi1/1 -> xps_library_ADCs_adc_user_datai1/1, Compare To Constant2/1, Compare To Constant4/1
  delayi4/1 -> delayi0/1
  conv7/1(Out1) -> q3/1
  xps_library_ADCs_adc_user_dataq3/1 -> conv7/1(In1)
  conv6/1(Out1) -> q2/1
  xps_library_ADCs_adc_user_dataq2/1 -> conv6/1(In1)
  conv5/1(Out1) -> q1/1
  xps_library_ADCs_adc_user_dataq1/1 -> conv5/1(In1)
  conv4/1(Out1) -> q0/1
  xps_library_ADCs_adc_user_dataq0/1 -> conv4/1(In1)
  conv3/1(Out1) -> i3/1
  conv2/1(Out1) -> i2/1
  conv1/1(Out1) -> i1/1
  conv/1(Out1) -> i0/1
  xps_library_ADCs_adc_user_sync0/1 -> sync0/1
  xps_library_ADCs_adc_user_outofrangei0/1 -> outofrangei0/1
  xps_library_ADCs_adc_user_datai3/1 -> conv3/1(In1)
  xps_library_ADCs_adc_user_datai2/1 -> conv2/1(In1)
  xps_library_ADCs_adc_user_datai1/1 -> conv1/1(In1)
  delayi11/1 -> delayq3/1
  delayi10/1 -> delayq2/1
  delayi9/1 -> delayq1/1
  delayi7/1 -> delayi3/1
  delayi6/1 -> delayi2/1
  delayi5/1 -> delayi1/1
  delayi0/1 -> xps_library_ADCs_adc_user_datai0/1, Compare To Constant/1, Compare To Constant3/1
  delayi8/1 -> delayq0/1
  delayq0/1 -> xps_library_ADCs_adc_user_dataq0/1, Compare To Constant11/1, Compare To Constant8/1
  xps_library_ADCs_adc_user_outofrangei1/1 -> outofrangei1/1
  Compare To Constant3/1 -> Logical Operator/1
  Compare To Constant/1 -> Logical Operator/2
  Compare To Constant4/1 -> Logical Operator/3
  Compare To Constant2/1 -> Logical Operator/4
  Logical Operator/1 -> xps_library_ADCs_adc_user_outofrangei0/1
  Compare To Constant6/1 -> Logical Operator1/1
  Compare To Constant1/1 -> Logical Operator1/2
  Compare To Constant7/1 -> Logical Operator1/3
  Compare To Constant5/1 -> Logical Operator1/4
  Logical Operator1/1 -> xps_library_ADCs_adc_user_outofrangei1/1
  xps_library_ADCs_adc_user_outofrangeq0/1 -> outofrangeq0/1
  xps_library_ADCs_adc_user_outofrangeq1/1 -> outofrangeq1/1
  Compare To Constant11/1 -> Logical Operator2/1
  Compare To Constant8/1 -> Logical Operator2/2
  Compare To Constant12/1 -> Logical Operator2/3
  Compare To Constant10/1 -> Logical Operator2/4
  Logical Operator2/1 -> xps_library_ADCs_adc_user_outofrangeq0/1
  Compare To Constant14/1 -> Logical Operator3/1
  Compare To Constant9/1 -> Logical Operator3/2
  Compare To Constant15/1 -> Logical Operator3/3
  Compare To Constant13/1 -> Logical Operator3/4
  Logical Operator3/1 -> xps_library_ADCs_adc_user_outofrangeq1/1
  sim_sync/1 -> delayi12/1, delayi13/1, delayi15/1, delayi14/1
  delayi14/1 -> delaysync0/1
  delayi15/1 -> delaysync1/1
  delaysync0/1 -> xps_library_ADCs_adc_user_sync0/1
  xps_library_ADCs_adc_user_sync1/1 -> sync1/1
  delayi12/1 -> delaysync2/1
  delayi13/1 -> delaysync3/1
  delaysync2/1 -> xps_library_ADCs_adc_user_sync2/1
  delaysync3/1 -> xps_library_ADCs_adc_user_sync3/1
  xps_library_ADCs_adc_user_sync2/1 -> sync2/1
  xps_library_ADCs_adc_user_sync3/1 -> sync3/1
  xps_library_ADCs_adc_user_data_valid/1 -> data_valid/1
  sim_data_valid/1 -> xps_library_ADCs_adc_user_data_valid/1
  xps_library_ADCs_adc_user_datai0/1 -> conv/1(In1)
  sim_in/1 -> gain/1
  gain/1 -> bias/1
  bias/1 -> delayi4/1, delayi5/1, delayi6/1, delayi7/1, delayi8/1, delayi11/1, delayi9/1, delayi10/1

== system xps_library/ADCs/adc16x250_8 ==
  a1_sim : Inport
  a2_sim : Inport  Port=2
  a3_sim : Inport  Port=3
  a4_sim : Inport  Port=4
  b1_sim : Inport  Port=5
  b2_sim : Inport  Port=6
  b3_sim : Inport  Port=7
  b4_sim : Inport  Port=8
  c1_sim : Inport  Port=9
  c2_sim : Inport  Port=10
  c3_sim : Inport  Port=11
  c4_sim : Inport  Port=12
  d1_sim : Inport  Port=13
  d2_sim : Inport  Port=14
  d3_sim : Inport  Port=15
  d4_sim : Inport  Port=16
  xps_library_ADCs_adc16x250_8_a{1..4} (4 alike) : xbsIndex_r4/Gateway In  gui_display_data_type=Fixed-point  arith_type="Signed  (2's comp)"  n_bits=8  bin_pt=7  preci_type=Single  exp_width=8  frac_width=24  rows=1  columns=1  quantization="Round  (unbiased: +/- Inf)"  overflow=Saturate  period=1  UseAsADC=off  ADCChannel='1'  interface=None  automatic_assignment=on  address_offset=hex2dec('00')  intf_name=''  intf_description=''  default_value=0  timing_constraint=None  locs_specified=off  LOCs={}  io_standard={}  inherit_from_input=off  hdl_port=on  dbl_ovrd=off  block_type=gatewayin
  xps_library_ADCs_adc16x250_8_b{1..4} (4 alike) : xbsIndex_r4/Gateway In  gui_display_data_type=Fixed-point  arith_type="Signed  (2's comp)"  n_bits=8  bin_pt=7  preci_type=Single  exp_width=8  frac_width=24  rows=1  columns=1  quantization="Round  (unbiased: +/- Inf)"  overflow=Saturate  period=1  UseAsADC=off  ADCChannel='1'  interface=None  automatic_assignment=on  address_offset=hex2dec('00')  intf_name=''  intf_description=''  default_value=0  timing_constraint=None  locs_specified=off  LOCs={}  io_standard={}  inherit_from_input=off  hdl_port=on  dbl_ovrd=off  block_type=gatewayin
  xps_library_ADCs_adc16x250_8_c{1..4} (4 alike) : xbsIndex_r4/Gateway In  gui_display_data_type=Fixed-point  arith_type="Signed  (2's comp)"  n_bits=8  bin_pt=7  preci_type=Single  exp_width=8  frac_width=24  rows=1  columns=1  quantization="Round  (unbiased: +/- Inf)"  overflow=Saturate  period=1  UseAsADC=off  ADCChannel='1'  interface=None  automatic_assignment=on  address_offset=hex2dec('00')  intf_name=''  intf_description=''  default_value=0  timing_constraint=None  locs_specified=off  LOCs={}  io_standard={}  inherit_from_input=off  hdl_port=on  dbl_ovrd=off  block_type=gatewayin
  xps_library_ADCs_adc16x250_8_d{1..4} (4 alike) : xbsIndex_r4/Gateway In  gui_display_data_type=Fixed-point  arith_type="Signed  (2's comp)"  n_bits=8  bin_pt=7  preci_type=Single  exp_width=8  frac_width=24  rows=1  columns=1  quantization="Round  (unbiased: +/- Inf)"  overflow=Saturate  period=1  UseAsADC=off  ADCChannel='1'  interface=None  automatic_assignment=on  address_offset=hex2dec('00')  intf_name=''  intf_description=''  default_value=0  timing_constraint=None  locs_specified=off  LOCs={}  io_standard={}  inherit_from_input=off  hdl_port=on  dbl_ovrd=off  block_type=gatewayin
  a1 : Outport
  a2 : Outport  Port=2
  a3 : Outport  Port=3
  a4 : Outport  Port=4
  b1 : Outport  Port=5
  b2 : Outport  Port=6
  b3 : Outport  Port=7
  b4 : Outport  Port=8
  c1 : Outport  Port=9
  c2 : Outport  Port=10
  c3 : Outport  Port=11
  c4 : Outport  Port=12
  d1 : Outport  Port=13
  d2 : Outport  Port=14
  d3 : Outport  Port=15
  d4 : Outport  Port=16
  wires:
  a1_sim/1 -> xps_library_ADCs_adc16x250_8_a1/1
  xps_library_ADCs_adc16x250_8_a1/1 -> a1/1  "a1"
  a2_sim/1 -> xps_library_ADCs_adc16x250_8_a2/1
  xps_library_ADCs_adc16x250_8_a2/1 -> a2/1  "a2"
  a3_sim/1 -> xps_library_ADCs_adc16x250_8_a3/1
  xps_library_ADCs_adc16x250_8_a3/1 -> a3/1  "a3"
  a4_sim/1 -> xps_library_ADCs_adc16x250_8_a4/1
  xps_library_ADCs_adc16x250_8_a4/1 -> a4/1  "a4"
  b1_sim/1 -> xps_library_ADCs_adc16x250_8_b1/1
  xps_library_ADCs_adc16x250_8_b1/1 -> b1/1  "b1"
  b2_sim/1 -> xps_library_ADCs_adc16x250_8_b2/1
  xps_library_ADCs_adc16x250_8_b2/1 -> b2/1  "b2"
  b3_sim/1 -> xps_library_ADCs_adc16x250_8_b3/1
  xps_library_ADCs_adc16x250_8_b3/1 -> b3/1  "b3"
  b4_sim/1 -> xps_library_ADCs_adc16x250_8_b4/1
  xps_library_ADCs_adc16x250_8_b4/1 -> b4/1  "b4"
  c1_sim/1 -> xps_library_ADCs_adc16x250_8_c1/1
  xps_library_ADCs_adc16x250_8_c1/1 -> c1/1  "c1"
  c2_sim/1 -> xps_library_ADCs_adc16x250_8_c2/1
  xps_library_ADCs_adc16x250_8_c2/1 -> c2/1  "c2"
  c3_sim/1 -> xps_library_ADCs_adc16x250_8_c3/1
  xps_library_ADCs_adc16x250_8_c3/1 -> c3/1  "c3"
  c4_sim/1 -> xps_library_ADCs_adc16x250_8_c4/1
  xps_library_ADCs_adc16x250_8_c4/1 -> c4/1  "c4"
  d1_sim/1 -> xps_library_ADCs_adc16x250_8_d1/1
  xps_library_ADCs_adc16x250_8_d1/1 -> d1/1  "d1"
  d2_sim/1 -> xps_library_ADCs_adc16x250_8_d2/1
  xps_library_ADCs_adc16x250_8_d2/1 -> d2/1  "d2"
  d3_sim/1 -> xps_library_ADCs_adc16x250_8_d3/1
  xps_library_ADCs_adc16x250_8_d3/1 -> d3/1  "d3"
  d4_sim/1 -> xps_library_ADCs_adc16x250_8_d4/1
  xps_library_ADCs_adc16x250_8_d4/1 -> d4/1  "d4"
